simulink model "SimulationBangBangHysteresisModel"  (R2024a)
settings: Solver=FixedStepAuto  StartTime=0.0  StopTime=tFinal_s  FixedStep=deltaT_s  RelTol=1e-3
values from neighbouring files (symbols this model uses):
  deadbandSize_C = 2    [Step02a_SimulationBangBangHysteresisSetupModel.m]
  K = 49    [Step01_SimulationBangBangSetupModel.m]    (also in Step02a_SimulationBangBangHysteresisSetupModel.m)
  Tambient_C = 24.1875    [Step01_SimulationBangBangSetupModel.m]    (also in Step02a_SimulationBangBangHysteresisSetupModel.m)
  u_ON = 1    [Step01_SimulationBangBangSetupModel.m]    (also in Step02a_SimulationBangBangHysteresisSetupModel.m)
libraries: TemperatureControlLibrary x4
settings Model: PacingRate=3  Creator=chris  LastModifiedBy=chris

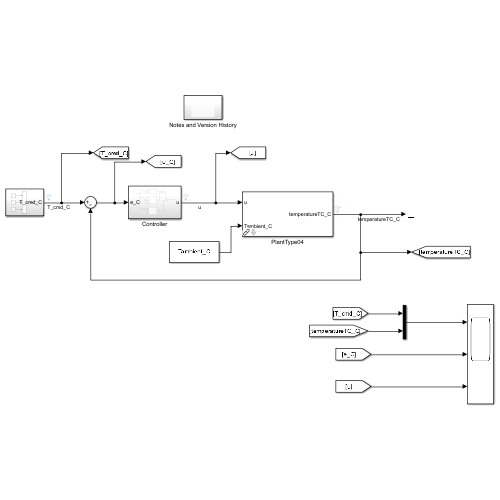
[thumbnail: Simulink's stored preview of the top-level diagram]
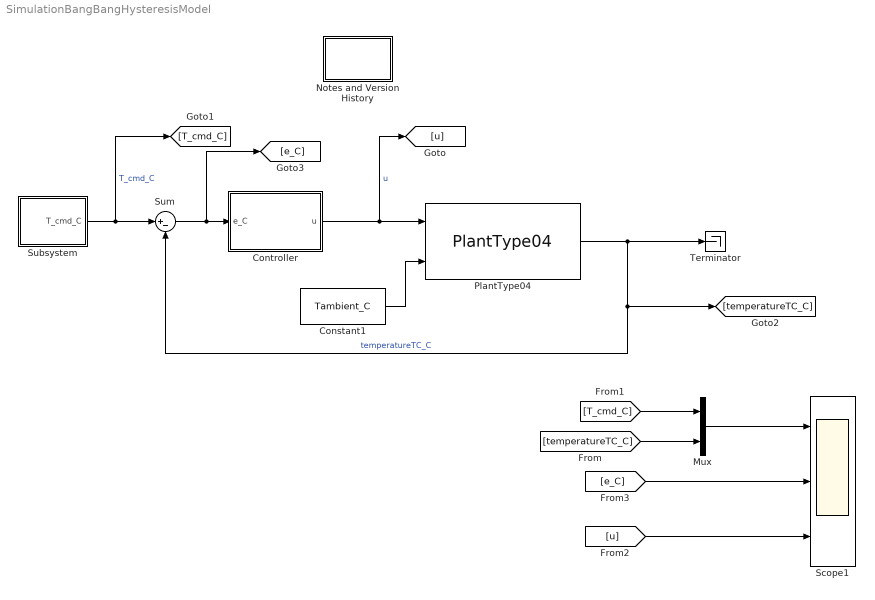
== system SimulationBangBangHysteresisModel ==
  Constant1 : Constant  Value=Tambient_C
  Controller : Subsystem
  Mux : Mux  Inputs=2
  Notes and Version History : Subsystem
  PlantType04 : TemperatureControlLibrary/PlantType04  wn=wn  zeta=zeta  K=K  Tdelay_s=Tdelay_s  noisePower=noisePower  Tsample_s=deltaT_s
  Scope1 : Scope  NumInputPorts=3
  Subsystem : Subsystem
  Sum : Sum  Inputs=|+-
  Terminator : Terminator
  wires:
  PlantType04/1 -> Terminator/1, [temperatureTC_C], Sum/2  "temperatureTC_C"
  Subsystem/1(T_cmd_C) -> [T_cmd_C], Sum/1  "T_cmd_C"
  Mux/1 -> Scope1/1
  [temperatureTC_C] -> Mux/2
  [T_cmd_C] -> Mux/1
  [u] -> Scope1/3
  Constant1/1 -> PlantType04/2
  Controller/1(u) -> PlantType04/1, [u]  "u"
  Sum/1 -> [e_C], Controller/1(e_C)
  [e_C] -> Scope1/2

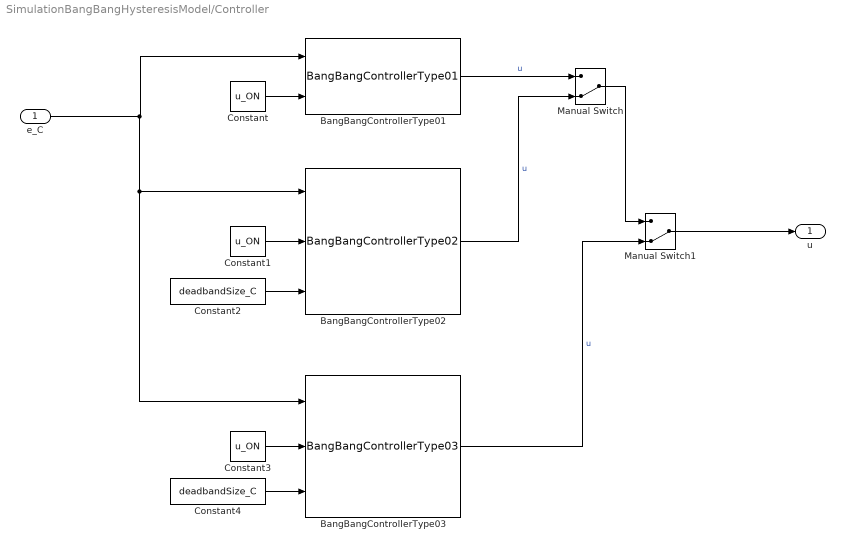
== system SimulationBangBangHysteresisModel/Controller ==
  e_C : Inport
  BangBangControllerType01 : TemperatureControlLibrary/BangBangControllerType01
  BangBangControllerType02 : TemperatureControlLibrary/BangBangControllerType02
  BangBangControllerType03 : TemperatureControlLibrary/BangBangControllerType03
  Constant : Constant  Value=u_ON
  Constant1 : Constant  Value=u_ON
  Constant2 : Constant  Value=deadbandSize_C
  Constant3 : Constant  Value=u_ON
  Constant4 : Constant  Value=deadbandSize_C
  Manual Switch : ManualSwitch  CurrentSetting=0
  Manual Switch1 : ManualSwitch  CurrentSetting=0
  u : Outport
  wires:
  Constant/1 -> BangBangControllerType01/2
  BangBangControllerType01/1 -> Manual Switch/1  "u"
  e_C/1 -> BangBangControllerType03/1, BangBangControllerType02/1, BangBangControllerType01/1
  Manual Switch/1 -> Manual Switch1/1
  Constant1/1 -> BangBangControllerType02/2
  Constant2/1 -> BangBangControllerType02/3
  BangBangControllerType02/1 -> Manual Switch/2  "u"
  Constant3/1 -> BangBangControllerType03/2
  Constant4/1 -> BangBangControllerType03/3
  BangBangControllerType03/1 -> Manual Switch1/2  "u"
  Manual Switch1/1 -> u/1

== system SimulationBangBangHysteresisModel/Notes and Version History ==
  note: Christopher Lum
      | lum@uw.edu
      |
      | Version History
      | 01/26/25: Created

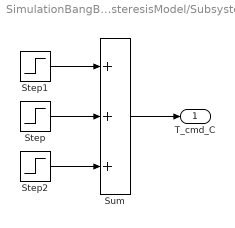
== system SimulationBangBangHysteresisModel/Subsystem ==
  Step : Step  Time=2.5*60  After=-5  SampleTime=0
  Step1 : Step  Time=5  After=45  SampleTime=0
  Step2 : Step  Time=250  After=10  SampleTime=0
  Sum : Sum  Inputs=+++
  T_cmd_C : Outport
  wires:
  Step2/1 -> Sum/3
  Sum/1 -> T_cmd_C/1
  Step/1 -> Sum/2
  Step1/1 -> Sum/1
